simulink model "dcdc_17b"  (R2017b)
settings: Solver=VariableStepAuto  StartTime=0.0  StopTime=0.08  FixedStep=t_step  MaxStep=1e-7  RelTol=1e-3
values from neighbouring files (symbols this model uses):
  Cb = (Vo-Vb)*T/2/Rb/delta_vo    (= 0.000141176470588)    [Buck_boost_voltage_control_design.m]    (also in buck_boost_tfs.m = 0.00130196078431)
  D = Vo/(Vs+Vo)    (= 0.498186215236)    [Buck_boost_voltage_control_design.m]    (also in buck_boost_tfs.m = 0.4)
  ki = 1e3    (= 1000)    [Buck_boost_voltage_control_design.m]    (also in buck_boost_tfs.m = 1)
  kp = 1    [Buck_boost_voltage_control_design.m]    (also in buck_boost_tfs.m = 0.005)
  Lb = (2*Rb*D*zeta)^2*Cb    [Buck_boost_voltage_control_design.m]    (also in buck_boost_tfs.m = 0.00195294117647)
  Vb = 400    [Buck_boost_voltage_control_design.m]    (also in buck_boost_tfs.m = 0)
  Vs = 415    [Buck_boost_voltage_control_design.m]    (also in buck_boost_tfs.m)
undefined symbols (not defined in the file or in its folder): Ion, Lithium, t_step
libraries: powerlib x23, powerlib_meascontrol x2, electricdrivelib x1
settings Model: Creator=Chuanyue Li  LastModifiedBy=c2107789
settings SolverCC: ZeroCrossAlgorithm=Adaptive
settings DebuggingCC: IgnoredZcDiagnostic=none

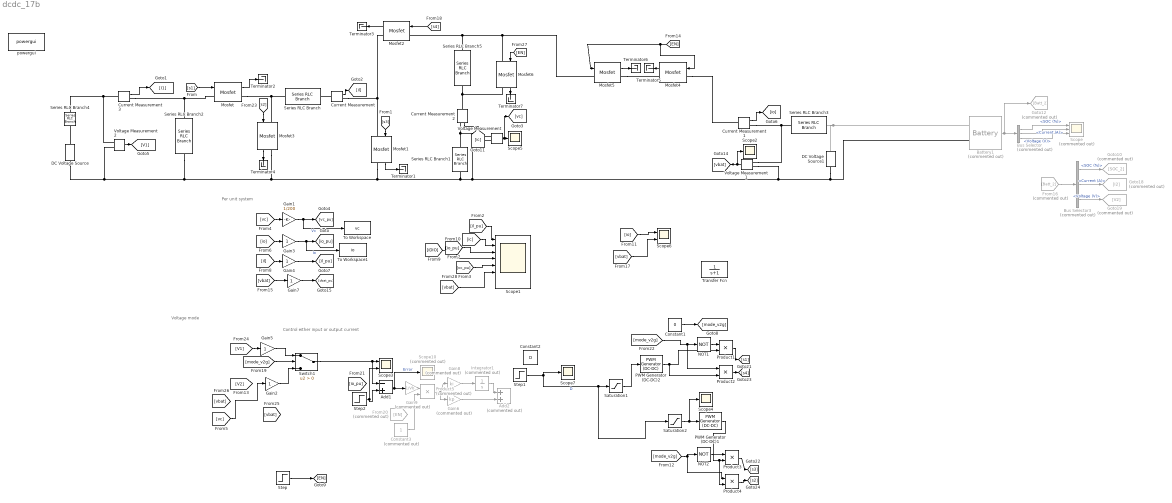
== system dcdc_17b ==
  note: Per unit system
  note: Control either input or output current
  note: Voltage mode
  Add1 : Sum  Inputs=-+
  Add2 : Sum  Commented=on
  Battery1 : electricdrivelib/Extra Sources/Battery  Commented=on  BatType=Lithium-Ion  ShowTempParam=off  ThermalPreset=no  ShowAgeParam=off  NomV=380  NomQ=500  SOC=69.98  Batt_Tr=1  PresetModel=on  MaxQ=500  MinV=285  FullV=442.3151  Dis_rate=217.3913  R=0.0076  Normal_OP=452.1739  expZone="[410.5466      24.56522]"  current=[6.5 13 32.5]  Units=Time  Tci=20  NomT=20  T2=-30  MaxQ2=4.8  FullV2=7.1  Normal_OP2=5.655  expZone2="[6.58           1]"  Rca=0.6  ti=2000  Dp=0  Neq0=0  Tsim=1e6  Ta1=25  Qeol=5.4*0.9  Reol=0.013333*1.2  Char_age=[2.3478, 3]  Dis_age=[2.3478, 10]  N1=1500  N2=10500  N3=1000  N4=1400  Ta2=45  N5=950
  Bus Selector : BusSelector  Commented=on  OutputSignals=SOC (%),Current (A),Voltage (V)
  Bus Selector3 : BusSelector  Commented=on  OutputSignals=SOC (%),Current (A),Voltage (V)
  Constant1 : Constant  Value=0
  Constant2 : Constant  Value=D
  Constant3 : Constant  Commented=on
  Current Measurement{,1..3} (4 alike) : powerlib/Measurements/Current Measurement  PhasorSimulation=off  OutputType=Complex  PSBequivalent=0
  DC Voltage Source : powerlib/Electrical Sources/DC Voltage Source  Amplitude=Vs  Measurements=None
  DC Voltage Source1 : powerlib/Electrical Sources/DC Voltage Source  Amplitude=Vb  Measurements=None
  From16 : From  Commented=on  GotoTag=Batt_2
  From20 : From  Commented=on  GotoTag=EN
  Gain1 : Gain  Gain=1/200
  Gain{2..5,7} (5 alike) : Gain
  Gain6 : Gain  Commented=on  Gain=kp
  Gain8 : Gain  Commented=on  Gain=ki
  Gain9 : Gain  Commented=on  Gain=1/Vb
  Goto10 : Goto  Commented=on  GotoTag=SOC_2
  Goto12 : Goto  Commented=on  GotoTag=Batt_2
  Goto18 : Goto  Commented=on  GotoTag=I2
  Goto19 : Goto  Commented=on  GotoTag=V2
  Integrator1 : Integrator  Commented=on  LimitOutput=on  UpperSaturationLimit=1  LowerSaturationLimit=0
  Mosfet{,2..6} (6 alike) : powerlib/Power Electronics/Mosfet  Ron=0.1  Lon=0  Rd=0.01  Vfd=0  IC=0  Rs=1e5  Cs=inf  Measurements=on
  Mosfet1 : powerlib/Power Electronics/Mosfet  Ron=0.01  Lon=0  Rd=0.01  Vfd=0  IC=0  Rs=1e5  Cs=inf  Measurements=on
  NOT1 : Logic  Operator=NOT  IconShape=distinctive  AllPortsSameDT=off  OutDataTypeStr=boolean
  NOT2 : Logic  Operator=NOT  IconShape=distinctive  AllPortsSameDT=off  OutDataTypeStr=boolean
  PWM Generator (DC-DC)1 : powerlib_meascontrol/Pulse & Signal Generators/PWM Generator (DC-DC)  Fsw=s_fre  Ts=0
  PWM Generator (DC-DC)2 : powerlib_meascontrol/Pulse & Signal Generators/PWM Generator (DC-DC)  Fsw=s_fre  Ts=0
  Product{1..4} (4 alike) : Product
  Product5 : Product  Commented=on
  Saturation1 : Saturate  UpperLimit=1  LowerLimit=0
  Saturation2 : Saturate  UpperLimit=0.95  LowerLimit=0
  Scope : Scope  Commented=on  NumInputPorts=3
  Scope1 : Scope  NumInputPorts=8
  Scope10 : Scope  Commented=on
  Scope{2,4..5,7} (4 alike) : Scope
  Scope3 : Scope  NumInputPorts=2
  Scope6 : Scope  NumInputPorts=2
  Series RLC Branch : powerlib/Elements/Series RLC Branch  LConnTagsString=__new0  RConnTagsString=__new0  BranchType=L  Resistance=1  Inductance=Lb  SetiL0=off  InitialCurrent=0  Capacitance=1e-6  Setx0=off  InitialVoltage=0  Measurements=None
  Series RLC Branch1 : powerlib/Elements/Series RLC Branch  LConnTagsString=__new0  RConnTagsString=__new0  BranchType=C  Resistance=1  Inductance=1e-3  SetiL0=off  InitialCurrent=0  Capacitance=Cb  Setx0=off  InitialVoltage=0  Measurements=None
  Series RLC Branch2 : powerlib/Elements/Series RLC Branch  LConnTagsString=__new0  RConnTagsString=__new0  BranchType=C  Resistance=1  Inductance=1e-3  SetiL0=off  InitialCurrent=0  Capacitance=Cb  Setx0=off  InitialVoltage=0  Measurements=None
  Series RLC Branch3 : powerlib/Elements/Series RLC Branch  LConnTagsString=__new0  RConnTagsString=__new0  BranchType=R  Resistance=1  Inductance=1e-3  SetiL0=off  InitialCurrent=0  Capacitance=Cb  Setx0=off  InitialVoltage=0  Measurements=None
  Series RLC Branch4 : powerlib/Elements/Series RLC Branch  LConnTagsString=__new0  RConnTagsString=__new0  BranchType=R  Resistance=1e-3  Inductance=1e-3  SetiL0=off  InitialCurrent=0  Capacitance=Cb  Setx0=off  InitialVoltage=0  Measurements=None
  Series RLC Branch5 : powerlib/Elements/Series RLC Branch  LConnTagsString=__new0  RConnTagsString=__new0  BranchType=R  Resistance=10  Inductance=Lb  SetiL0=off  InitialCurrent=0  Capacitance=1e-6  Setx0=off  InitialVoltage=0  Measurements=None
  Step : Step  Time=0.01  SampleTime=0
  Step1 : Step  Time=0.04  Before=D  After=D+0.05  SampleTime=0
  Step2 : Step  Time=0.2  Before=405  After=410  SampleTime=0
  Switch1 : Switch  Criteria=u2 > Threshold
  Terminator{1..7} (7 alike) : Terminator
  To Workspace : ToWorkspace  VariableName=vc  SaveFormat=Timeseries  SampleTime=-1
  To Workspace1 : ToWorkspace  VariableName=io  SaveFormat=Timeseries  SampleTime=-1
  Transfer Fcn : TransferFcn  Denominator=[1 1]
  Voltage Measurement : powerlib/Measurements/Voltage Measurement  PhasorSimulation=off  OutputType=Complex  PSBequivalent=0
  Voltage Measurement1 : powerlib/Measurements/Voltage Measurement  PhasorSimulation=off  OutputType=Complex  PSBequivalent=0
  Voltage Measurement2 : powerlib/Measurements/Voltage Measurement  PhasorSimulation=off  OutputType=Complex  PSBequivalent=0
  powergui : powerlib/powergui  Priority=1  SimulationMode=Continuous  SampleTime=t_step*10  frequency=60  Iterations=50  frequencyindice=0  Pbase=100e6  ErrMax=1e-4  UnitsV=kV  UnitsW=MW  buscounter=0  FunctionMessages=off  echomessages=off  EnableUseOfTLC=off  CurrentSourceSwitches=off  DisableSnubberDevices=off  DisableRonSwitches=off  DisableVfSwitches=off  DisplayEquations=off  AutomaticDiscreteSolvers=off  SolverType=Tustin/Backward Euler (TBE)  Interpol=off  ExternalGateDelay=off  methode=off  Ts=100  x0status=blocks  SPID=off  SwTol=0  HookPort=off  NonlinearTolerance=1e-4  nMaxIteration=100  ContinueOnMaxIteration=off  RestoreLinks=warning  ResistiveCurrentMeasurement=off  Frange=[0:2:500]  Ylog=off  Xlog=on  ShowGrid=off  save=off  variable=ZData  structure=0  ZoomFFT=off  StartTime=0.0  cycles=1  DisplayStyle=1  fundamental=60  FreqAxis=off  MaxFrequency=1000  frequencyindicesteady=1  RmsSteady=1  display=off
  wires:
  [s1] -> Mosfet/1
  [s3] -> Mosfet1/1
  Current Measurement/1 -> [il]
  Voltage Measurement/1 -> Scope5/1, [vc]
  [il_pu] -> Scope1/1
  [vc] -> Gain1/1
  Gain1/1 -> To Workspace/1, [vc_pu]  "Vc"
  Bus Selector/1 -> Scope/1  "<SOC (%)>"
  Bus Selector/2 -> Scope/2  "<Current (A)>"
  Bus Selector/3 -> Scope/3  "<Voltage (V)>"
  [io] -> Gain3/1
  Current Measurement1/1 -> [io]
  Gain3/1 -> To Workspace1/1, [io_pu]  "Io"
  [io_pu] -> Scope1/3
  Gain4/1 -> [il_pu]
  [il] -> Gain4/1
  [iDIO] -> Scope1/4
  Current Measurement2/1 -> [ic]
  [ic] -> Scope1/2
  [vc_pu] -> Scope1/5
  Voltage Measurement1/1 -> Scope2/1, [vbat]
  [vbat] -> Gain7/1
  Gain7/1 -> [vbat_pu]
  Mosfet1/1 -> Terminator1/1
  Mosfet/1 -> Terminator2/1
  Mosfet2/1 -> Terminator3/1
  [s4] -> Mosfet2/1
  [s2] -> Mosfet3/1
  Mosfet3/1 -> Terminator4/1
  Battery1/1 -> Goto12/1, Bus Selector/1
  From16/1 -> Bus Selector3/1
  Bus Selector3/3 -> Goto19/1  "<Voltage (V)>"
  Bus Selector3/2 -> Goto18/1  "<Current (A)>"
  Bus Selector3/1 -> Goto10/1  "<SOC (%)>"
  Current Measurement3/1 -> [I1]
  Voltage Measurement2/1 -> [V1]
  Switch1/1 -> Scope3/1, Add1/1
  Constant1/1 -> [mode_v2g]
  PWM Generator (DC-DC)1/1 -> Product3/2, Product4/2
  Product3/1 -> [s3]
  Product4/1 -> [s2]
  [mode_v2g] -> Product4/1, NOT2/1
  [mode_v2g] -> NOT1/1, Product2/1
  Product2/1 -> [s4]
  Product1/1 -> [s1]
  [mode_v2g] -> Switch1/2
  [vc] -> Gain2/1
  PWM Generator (DC-DC)2/1 -> Product2/2, Product1/2
  Saturation2/1 -> Scope4/1, PWM Generator (DC-DC)1/1
  Add1/1 -> Gain9/1, Scope10/1  "Error"
  Step2/1 -> Add1/2, Scope3/2
  Gain8/1 -> Integrator1/1
  Gain6/1 -> Add2/2
  Product5/1 -> Gain6/1, Gain8/1
  Constant3/1 -> Product5/2
  Step1/1 -> Saturation1/1, Saturation2/1, Scope7/1  "D"
  Integrator1/1 -> Add2/1
  Saturation1/1 -> PWM Generator (DC-DC)2/1
  NOT1/1 -> Product1/1
  NOT2/1 -> Product3/1
  Gain2/1 -> Switch1/3
  Gain5/1 -> Switch1/1
  [V1] -> Gain5/1
  Gain9/1 -> Product5/1
  Mosfet4/1 -> Terminator5/1
  Mosfet5/1 -> Terminator6/1
  [EN] -> Mosfet4/1, Mosfet5/1
  Step/1 -> [EN]
  Mosfet6/1 -> Terminator7/1
  [EN] -> Mosfet6/1
  [vbat] -> Scope1/6
  [io] -> Scope6/1
  [vbat] -> Scope6/2
  connections:
  Mosfet/RConn1 -- Mosfet3/LConn1 -- Series RLC Branch/LConn1
  Current Measurement/LConn1 -- Series RLC Branch/RConn1
  Current Measurement2/RConn1 -- Voltage Measurement/LConn1 -- Series RLC Branch1/LConn1
  Voltage Measurement/LConn2 -- Voltage Measurement2/LConn2 -- DC Voltage Source/LConn1 -- Series RLC Branch2/RConn1 -- Mosfet3/RConn1 -- Mosfet1/RConn1 -- Series RLC Branch1/RConn1 -- Voltage Measurement1/LConn2 -- DC Voltage Source1/LConn1 -- Battery1/LConn2
  Mosfet1/LConn1 -- Mosfet2/RConn1 -- Current Measurement/RConn1
  DC Voltage Source/RConn1 -- Series RLC Branch4/RConn1
  Current Measurement3/RConn1 -- Mosfet/LConn1 -- Series RLC Branch2/LConn1
  Series RLC Branch4/LConn1 -- Voltage Measurement2/LConn1 -- Current Measurement3/LConn1
  Voltage Measurement1/LConn1 -- Current Measurement1/RConn1 -- Series RLC Branch3/RConn1
  Battery1/LConn1 -- DC Voltage Source1/RConn1 -- Series RLC Branch3/LConn1
  Mosfet6/LConn1 -- Mosfet5/LConn1 -- Series RLC Branch5/LConn1 -- Mosfet2/LConn1
  Mosfet5/RConn1 -- Mosfet4/RConn1
  Mosfet6/RConn1 -- Series RLC Branch5/RConn1 -- Current Measurement2/LConn1
  Mosfet4/LConn1 -- Current Measurement1/LConn1
